simulink library "rwa_power_lib"  (R2018b)
settings: Solver=VariableStepAuto  StartTime=0.0  StopTime=10.0  RelTol=1e-3
undefined symbols (not defined in the file): simParams
settings Model: Creator=colem  LastModifiedBy=colem

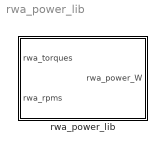
== system rwa_power_lib ==
  rwa_power_lib : Subsystem

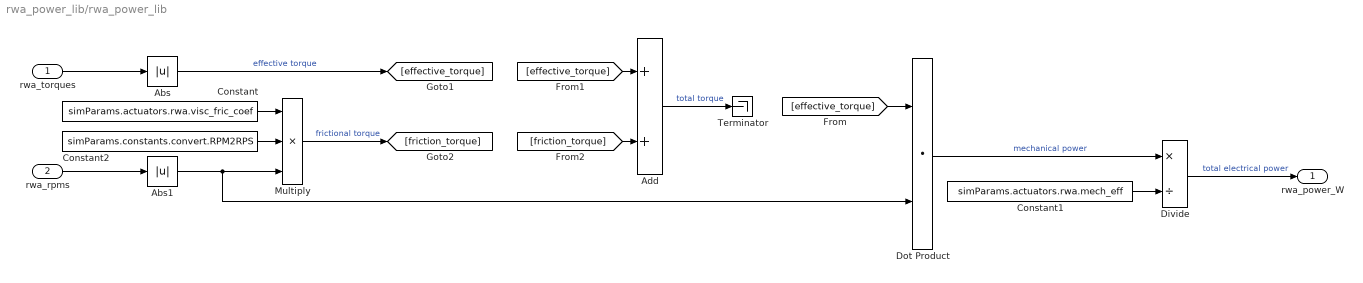
== system rwa_power_lib/rwa_power_lib ==
  rwa_torques : Inport
  rwa_rpms : Inport  Port=2
  Abs : Abs
  Abs1 : Abs
  Add : Sum
  Constant : Constant  Value=simParams.actuators.rwa.visc_fric_coef  SampleTime=simParams.sample_time_s
  Constant1 : Constant  Value=simParams.actuators.rwa.mech_eff  SampleTime=simParams.sample_time_s
  Constant2 : Constant  Value=simParams.constants.convert.RPM2RPS
  Divide : Product  Inputs=*/
  Dot Product : DotProduct  InputSameDT=on  OutDataTypeStr=Inherit: Inherit via internal rule
  Multiply : Product  Inputs=3
  Terminator : Terminator
  rwa_power_W : Outport
  wires:
  Multiply/1 -> [friction_torque]  "frictional torque"
  Add/1 -> Terminator/1  "total torque"
  Abs/1 -> [effective_torque]  "effective torque"
  Dot Product/1 -> Divide/1  "mechanical power"
  Constant/1 -> Multiply/1
  Abs1/1 -> Dot Product/2, Multiply/3
  Divide/1 -> rwa_power_W/1  "total electrical power"
  Constant1/1 -> Divide/2
  rwa_rpms/1 -> Abs1/1
  rwa_torques/1 -> Abs/1
  Constant2/1 -> Multiply/2
  [effective_torque] -> Dot Product/1
  [effective_torque] -> Add/1
  [friction_torque] -> Add/2
